simulink model "P702_NI_SoftECU"  (R2019a)
settings: Solver=ode1  StartTime=0.0  StopTime=Inf  FixedStep=0.001  RelTol=1e-3  EnableMultiTasking=on
PreLoadFcn:
  | run '.\VeriStand_BlockSet\NIVeriStandAddPaths.m'
undefined symbols (not defined in the file or in its folder): magnitude
libraries: simulink x83, simulink_extras x1
(part 65 of 76)

== system P702_NI_SoftECU/Output/Subsystem1/CAN_Signal/ECM_DIESEL PCM PCM_HEV/EngBrakeData_0x165 ==
  in_port : Inport
  AccEngStat_D_Actl : Terminator
  AccStopMde_D_Rq : Terminator
  BPedDrvAppl_D_QF : Terminator
  BpedDrvAppl_D_Actl : Terminator
  CcMde_D_Actl : Terminator
  CcOvrrdActv_B_Actl : Terminator
  CcStat_D_Actl : Terminator
  CmbbDeny_B_ActlPrpl : Terminator
  CmbbEngTqMn_B_Actl : Terminator
  EngAout_N_MnAllw : Terminator
  PrplTqMnSat_B_Actl : Terminator
  Veh_V_DsplyCcSet : Terminator
  bus_selector : BusSelector  OutputSignals=CmbbEngTqMn_B_Actl,CcOvrrdActv_B_Actl,BpedDrvAppl_D_Actl,CmbbDeny_B_ActlPrpl,AccEngStat_D_Actl,BPedDrvAppl_D_QF,CcMde_D_Actl,CcStat_D_Actl,Veh_V_DsplyCcSet,AccStopMde_D_Rq,PrplTqMnSat_B_Actl,EngAout_N_MnAllw
  wires:
  in_port/1 -> bus_selector/1  "Subsystem1"
  bus_selector/1 -> CmbbEngTqMn_B_Actl/1  "<CmbbEngTqMn_B_Actl>"
  bus_selector/2 -> CcOvrrdActv_B_Actl/1  "<CcOvrrdActv_B_Actl>"
  bus_selector/3 -> BpedDrvAppl_D_Actl/1  "<BpedDrvAppl_D_Actl>"
  bus_selector/4 -> CmbbDeny_B_ActlPrpl/1  "<CmbbDeny_B_ActlPrpl>"
  bus_selector/5 -> AccEngStat_D_Actl/1  "<AccEngStat_D_Actl>"
  bus_selector/6 -> BPedDrvAppl_D_QF/1  "<BPedDrvAppl_D_QF>"
  bus_selector/7 -> CcMde_D_Actl/1  "<CcMde_D_Actl>"
  bus_selector/8 -> CcStat_D_Actl/1  "<CcStat_D_Actl>"
  bus_selector/9 -> Veh_V_DsplyCcSet/1  "<Veh_V_DsplyCcSet>"
  bus_selector/10 -> AccStopMde_D_Rq/1  "<AccStopMde_D_Rq>"
  bus_selector/11 -> PrplTqMnSat_B_Actl/1  "<PrplTqMnSat_B_Actl>"
  bus_selector/12 -> EngAout_N_MnAllw/1  "<EngAout_N_MnAllw>"

== system P702_NI_SoftECU/Output/Subsystem1/CAN_Signal/ECM_DIESEL PCM PCM_HEV/EngVehicleSpThrottle2_0x202 ==
  in_port : Inport
  GearRvrse_D_Actl : Terminator
  StrtrMtrCtlMsgTxt_D2_Rq : Terminator
  StrtrMtrCtlMsgTxt_D_Rq : Terminator
  StrtrMtrDlyStrt_B_Stat : Terminator
  VehVActlEng_D_Qf : Terminator
  VehVActlEng_No_Cnt : Terminator
  VehVActlEng_No_Cs : Terminator
  VehVTrlrAid_B_Avail : Terminator
  Veh_V_ActlEng : Terminator
  Veh_V_RqCcSet : Terminator
  bus_selector : BusSelector  OutputSignals=StrtrMtrCtlMsgTxt_D_Rq,GearRvrse_D_Actl,StrtrMtrCtlMsgTxt_D2_Rq,VehVActlEng_No_Cs,VehVTrlrAid_B_Avail,VehVActlEng_No_Cnt,StrtrMtrDlyStrt_B_Stat,VehVActlEng_D_Qf,Veh_V_RqCcSet,Veh_V_ActlEng
  wires:
  in_port/1 -> bus_selector/1  "Subsystem1"
  bus_selector/1 -> StrtrMtrCtlMsgTxt_D_Rq/1  "<StrtrMtrCtlMsgTxt_D_Rq>"
  bus_selector/2 -> GearRvrse_D_Actl/1  "<GearRvrse_D_Actl>"
  bus_selector/3 -> StrtrMtrCtlMsgTxt_D2_Rq/1  "<StrtrMtrCtlMsgTxt_D2_Rq>"
  bus_selector/4 -> VehVActlEng_No_Cs/1  "<VehVActlEng_No_Cs>"
  bus_selector/5 -> VehVTrlrAid_B_Avail/1  "<VehVTrlrAid_B_Avail>"
  bus_selector/6 -> VehVActlEng_No_Cnt/1  "<VehVActlEng_No_Cnt>"
  bus_selector/7 -> StrtrMtrDlyStrt_B_Stat/1  "<StrtrMtrDlyStrt_B_Stat>"
  bus_selector/8 -> VehVActlEng_D_Qf/1  "<VehVActlEng_D_Qf>"
  bus_selector/9 -> Veh_V_RqCcSet/1  "<Veh_V_RqCcSet>"
  bus_selector/10 -> Veh_V_ActlEng/1  "<Veh_V_ActlEng>"

== system P702_NI_SoftECU/Output/Subsystem1/CAN_Signal/ECM_DIESEL PCM PCM_HEV/EngVehicleSpThrottle_0x204 ==
  in_port : Inport
  ApedPosPcActl_D_Qf : Terminator
  ApedPosPcActl_No_Cnt : Terminator
  ApedPosPcActl_No_Cs : Terminator
  ApedPos_PcRate_ActlArb : Terminator
  ApedPos_Pc_ActlArb : Terminator
  EngAout3_N_Actl : Terminator
  EngAoutNActl_D_QF : Terminator
  EngAout_N_Actl : Terminator
  bus_selector : BusSelector  OutputSignals=ApedPosPcActl_D_Qf,ApedPosPcActl_No_Cnt,ApedPos_Pc_ActlArb,ApedPos_PcRate_ActlArb,EngAoutNActl_D_QF,EngAout_N_Actl,ApedPosPcActl_No_Cs,EngAout3_N_Actl
  wires:
  in_port/1 -> bus_selector/1  "Subsystem1"
  bus_selector/1 -> ApedPosPcActl_D_Qf/1  "<ApedPosPcActl_D_Qf>"
  bus_selector/2 -> ApedPosPcActl_No_Cnt/1  "<ApedPosPcActl_No_Cnt>"
  bus_selector/3 -> ApedPos_Pc_ActlArb/1  "<ApedPos_Pc_ActlArb>"
  bus_selector/4 -> ApedPos_PcRate_ActlArb/1  "<ApedPos_PcRate_ActlArb>"
  bus_selector/5 -> EngAoutNActl_D_QF/1  "<EngAoutNActl_D_QF>"
  bus_selector/6 -> EngAout_N_Actl/1  "<EngAout_N_Actl>"
  bus_selector/7 -> ApedPosPcActl_No_Cs/1  "<ApedPosPcActl_No_Cs>"
  bus_selector/8 -> EngAout3_N_Actl/1  "<EngAout3_N_Actl>"

== system P702_NI_SoftECU/Output/Subsystem1/CAN_Signal/ECM_DIESEL PCM PCM_HEV/EngineClimateData_0x178 ==
  in_port : Inport
  AirAmbTe_D_Qf : Terminator
  AirAmb_P_Actl : Terminator
  AirAmb_Te_Actl : Terminator
  AirAmb_Te_ActlFilt : Terminator
  AslChime_B_Rq : Terminator
  AslIconDsply_D_Rq : Terminator
  DynoMde_B_Cmd : Terminator
  EcssLamp_D_RqDsply : Terminator
  EngAout_Aa_Actl : Terminator
  GasPrtc_D_RqDsply : Terminator
  HvacHtrCore2_Te_Actl : Terminator
  bus_selector : BusSelector  OutputSignals=DynoMde_B_Cmd,AslIconDsply_D_Rq,HvacHtrCore2_Te_Actl,GasPrtc_D_RqDsply,EcssLamp_D_RqDsply,EngAout_Aa_Actl,AslChime_B_Rq,AirAmbTe_D_Qf,AirAmb_Te_Actl,AirAmb_P_Actl,AirAmb_Te_ActlFilt
  wires:
  in_port/1 -> bus_selector/1  "Subsystem1"
  bus_selector/1 -> DynoMde_B_Cmd/1  "<DynoMde_B_Cmd>"
  bus_selector/2 -> AslIconDsply_D_Rq/1  "<AslIconDsply_D_Rq>"
  bus_selector/3 -> HvacHtrCore2_Te_Actl/1  "<HvacHtrCore2_Te_Actl>"
  bus_selector/4 -> GasPrtc_D_RqDsply/1  "<GasPrtc_D_RqDsply>"
  bus_selector/5 -> EcssLamp_D_RqDsply/1  "<EcssLamp_D_RqDsply>"
  bus_selector/6 -> EngAout_Aa_Actl/1  "<EngAout_Aa_Actl>"
  bus_selector/7 -> AslChime_B_Rq/1  "<AslChime_B_Rq>"
  bus_selector/8 -> AirAmbTe_D_Qf/1  "<AirAmbTe_D_Qf>"
  bus_selector/9 -> AirAmb_Te_Actl/1  "<AirAmb_Te_Actl>"
  bus_selector/10 -> AirAmb_P_Actl/1  "<AirAmb_P_Actl>"
  bus_selector/11 -> AirAmb_Te_ActlFilt/1  "<AirAmb_Te_ActlFilt>"

== system P702_NI_SoftECU/Output/Subsystem1/CAN_Signal/ECM_DIESEL PCM PCM_HEV/EngineData_6_0x156 ==
  in_port : Inport
  EngClntTe_D_Qf : Terminator
  EngClnt_Te_Actl : Terminator
  EngGoutLss_Tq_Est : Terminator
  EngOil_Te_Actl : Terminator
  EngOvrhtMitgActv_D_Ind : Terminator
  bus_selector : BusSelector  OutputSignals=EngClnt_Te_Actl,EngOil_Te_Actl,EngGoutLss_Tq_Est,EngOvrhtMitgActv_D_Ind,EngClntTe_D_Qf
  wires:
  in_port/1 -> bus_selector/1  "Subsystem1"
  bus_selector/1 -> EngClnt_Te_Actl/1  "<EngClnt_Te_Actl>"
  bus_selector/2 -> EngOil_Te_Actl/1  "<EngOil_Te_Actl>"
  bus_selector/3 -> EngGoutLss_Tq_Est/1  "<EngGoutLss_Tq_Est>"
  bus_selector/4 -> EngOvrhtMitgActv_D_Ind/1  "<EngOvrhtMitgActv_D_Ind>"
  bus_selector/5 -> EngClntTe_D_Qf/1  "<EngClntTe_D_Qf>"

== system P702_NI_SoftECU/Output/Subsystem1/CAN_Signal/ECM_DIESEL PCM PCM_HEV/EngineData_7_0x179 ==
  in_port : Inport
  AirCondClutch_B_Stats : Terminator
  AirCondRec_B_Rq : Terminator
  EngOilLife_Pc_Actl : Terminator
  EngSrvcRqd_B_Rq : Terminator
  FuelFillInlet_B_Dsply : Terminator
  FuelFilterLamp_B_Dsply : Terminator
  FuelFlw_Vl_Dsply : Terminator
  HvacAirFullOut_B_Rq : Terminator
  OdoCount : Terminator
  TrnKickDown_B_RqDrv : Terminator
  TrnManShifGear_D_IndDrv : Terminator
  TrnManShif_D_IndDrv : Terminator
  bus_selector : BusSelector  OutputSignals=TrnManShif_D_IndDrv,HvacAirFullOut_B_Rq,TrnKickDown_B_RqDrv,EngSrvcRqd_B_Rq,EngOilLife_Pc_Actl,FuelFillInlet_B_Dsply,OdoCount,AirCondRec_B_Rq,TrnManShifGear_D_IndDrv,AirCondClutch_B_Stats,FuelFilterLamp_B_Dsply,FuelFlw_Vl_Dsply
  wires:
  in_port/1 -> bus_selector/1  "Subsystem1"
  bus_selector/1 -> TrnManShif_D_IndDrv/1  "<TrnManShif_D_IndDrv>"
  bus_selector/2 -> HvacAirFullOut_B_Rq/1  "<HvacAirFullOut_B_Rq>"
  bus_selector/3 -> TrnKickDown_B_RqDrv/1  "<TrnKickDown_B_RqDrv>"
  bus_selector/4 -> EngSrvcRqd_B_Rq/1  "<EngSrvcRqd_B_Rq>"
  bus_selector/5 -> EngOilLife_Pc_Actl/1  "<EngOilLife_Pc_Actl>"
  bus_selector/6 -> FuelFillInlet_B_Dsply/1  "<FuelFillInlet_B_Dsply>"
  bus_selector/7 -> OdoCount/1  "<OdoCount>"
  bus_selector/8 -> AirCondRec_B_Rq/1  "<AirCondRec_B_Rq>"
  bus_selector/9 -> TrnManShifGear_D_IndDrv/1  "<TrnManShifGear_D_IndDrv>"
  bus_selector/10 -> AirCondClutch_B_Stats/1  "<AirCondClutch_B_Stats>"
  bus_selector/11 -> FuelFilterLamp_B_Dsply/1  "<FuelFilterLamp_B_Dsply>"
  bus_selector/12 -> FuelFlw_Vl_Dsply/1  "<FuelFlw_Vl_Dsply>"

== system P702_NI_SoftECU/Output/Subsystem1/CAN_Signal/ECM_DIESEL PCM PCM_HEV/Engine_Clutch_Data_0x42F ==
  in_port : Inport
  CluPdlPosPcMeas_D_Qf : Terminator
  CluPdlPos_Pc_Meas : Terminator
  CluPdl_PcRate_Actl : Terminator
  EngAoutIdl_N_Ntrl : Terminator
  EngAout_N_Dsply : Terminator
  bus_selector : BusSelector  OutputSignals=CluPdl_PcRate_Actl,CluPdlPosPcMeas_D_Qf,CluPdlPos_Pc_Meas,EngAoutIdl_N_Ntrl,EngAout_N_Dsply
  wires:
  in_port/1 -> bus_selector/1  "Subsystem1"
  bus_selector/1 -> CluPdl_PcRate_Actl/1  "<CluPdl_PcRate_Actl>"
  bus_selector/2 -> CluPdlPosPcMeas_D_Qf/1  "<CluPdlPosPcMeas_D_Qf>"
  bus_selector/3 -> CluPdlPos_Pc_Meas/1  "<CluPdlPos_Pc_Meas>"
  bus_selector/4 -> EngAoutIdl_N_Ntrl/1  "<EngAoutIdl_N_Ntrl>"
  bus_selector/5 -> EngAout_N_Dsply/1  "<EngAout_N_Dsply>"

== system P702_NI_SoftECU/Output/Subsystem1/CAN_Signal/ECM_DIESEL PCM PCM_HEV/Gear_Shift_by_Wire_3 ==
  in_port : Inport
  GearSelLck_D_Rq : Terminator
  PrkBrkActv_D_RqTrnGear : Terminator
  TrnCmdCnt_B_Actl : Terminator
  TrnCmdState_B_Actl : Terminator
  TrnDtpCmd_D_Actl : Terminator
  TrnGearCmd_No_Cnt : Terminator
  TrnGearCmd_No_Cs : Terminator
  TrnGearCmd_Pc_ActlPt : Terminator
  TrnGearMsgTxt_D_Rq : Terminator
  TrnGearNtmAllow_B_Stat : Terminator
  TrnGear_D_RqPt : Terminator
  TrnLvrV_D_Rq : Terminator
  TrnNtrlTowCmd_D_Actl : Terminator
  TrnSbwSysHlth_D_Actl : Terminator
  TrnValidGear_D_Cnfm : Terminator
  bus_selector : BusSelector  OutputSignals=GearSelLck_D_Rq,PrkBrkActv_D_RqTrnGear,TrnCmdCnt_B_Actl,TrnCmdState_B_Actl,TrnDtpCmd_D_Actl,TrnGearCmd_No_Cnt,TrnGearCmd_No_Cs,TrnGearCmd_Pc_ActlPt,TrnGearMsgTxt_D_Rq,TrnGearNtmAllow_B_Stat,TrnGear_D_RqPt,TrnLvrV_D_Rq,TrnNtrlTowCmd_D_Actl,TrnSbwSysHlth_D_Actl,TrnValidGear_D_Cnfm
  wires:
  in_port/1 -> bus_selector/1  "Subsystem1"
  bus_selector/1 -> GearSelLck_D_Rq/1  "<GearSelLck_D_Rq>"
  bus_selector/2 -> PrkBrkActv_D_RqTrnGear/1  "<PrkBrkActv_D_RqTrnGear>"
  bus_selector/3 -> TrnCmdCnt_B_Actl/1  "<TrnCmdCnt_B_Actl>"
  bus_selector/4 -> TrnCmdState_B_Actl/1  "<TrnCmdState_B_Actl>"
  bus_selector/5 -> TrnDtpCmd_D_Actl/1  "<TrnDtpCmd_D_Actl>"
  bus_selector/6 -> TrnGearCmd_No_Cnt/1  "<TrnGearCmd_No_Cnt>"
  bus_selector/7 -> TrnGearCmd_No_Cs/1  "<TrnGearCmd_No_Cs>"
  bus_selector/8 -> TrnGearCmd_Pc_ActlPt/1  "<TrnGearCmd_Pc_ActlPt>"
  bus_selector/9 -> TrnGearMsgTxt_D_Rq/1  "<TrnGearMsgTxt_D_Rq>"
  bus_selector/10 -> TrnGearNtmAllow_B_Stat/1  "<TrnGearNtmAllow_B_Stat>"
  bus_selector/11 -> TrnGear_D_RqPt/1  "<TrnGear_D_RqPt>"
  bus_selector/12 -> TrnLvrV_D_Rq/1  "<TrnLvrV_D_Rq>"
  bus_selector/13 -> TrnNtrlTowCmd_D_Actl/1  "<TrnNtrlTowCmd_D_Actl>"
  bus_selector/14 -> TrnSbwSysHlth_D_Actl/1  "<TrnSbwSysHlth_D_Actl>"
  bus_selector/15 -> TrnValidGear_D_Cnfm/1  "<TrnValidGear_D_Cnfm>"

== system P702_NI_SoftECU/Output/Subsystem1/CAN_Signal/ECM_DIESEL PCM PCM_HEV/Global_PATS_TargetInfo_0x47 ==
  in_port : Inport
  bus_selector : BusSelector  OutputSignals=immoTarget1Status,immoTarget1Cmd,immoTarget1Data
  immoTarget1Cmd : Terminator
  immoTarget1Data : Terminator
  immoTarget1Status : Terminator
  wires:
  in_port/1 -> bus_selector/1  "Subsystem1"
  bus_selector/1 -> immoTarget1Status/1  "<immoTarget1Status>"
  bus_selector/2 -> immoTarget1Cmd/1  "<immoTarget1Cmd>"
  bus_selector/3 -> immoTarget1Data/1  "<immoTarget1Data>"

== system P702_NI_SoftECU/Output/Subsystem1/CAN_Signal/ECM_DIESEL PCM PCM_HEV/HEV_Powertrain_Data2 ==
  in_port : Inport
  BattTracCnnct_D_Rq : Terminator
  PrplTqMnRgen_B_Actl : Terminator
  WhlDirAvgDrv_D_Actl : Terminator
  bus_selector : BusSelector  OutputSignals=BattTracCnnct_D_Rq,PrplTqMnRgen_B_Actl,WhlDirAvgDrv_D_Actl
  wires:
  in_port/1 -> bus_selector/1  "Subsystem1"
  bus_selector/1 -> BattTracCnnct_D_Rq/1  "<BattTracCnnct_D_Rq>"
  bus_selector/2 -> PrplTqMnRgen_B_Actl/1  "<PrplTqMnRgen_B_Actl>"
  bus_selector/3 -> WhlDirAvgDrv_D_Actl/1  "<WhlDirAvgDrv_D_Actl>"

== system P702_NI_SoftECU/Output/Subsystem1/CAN_Signal/ECM_DIESEL PCM PCM_HEV/PCM_AutoSar_NetworkMgmt_0x595 ==
  in_port : Inport
  PCM_AutoSarNMControl : Terminator
  PCM_AutoSarNMNodeId : Terminator
  PCM_AutoSarNMReserved{1..4} (4 alike) : Terminator
  PCM_GWNMProxy : Terminator
  PCM_GWOnBoardTester : Terminator
  bus_selector : BusSelector  OutputSignals=PCM_AutoSarNMNodeId,PCM_AutoSarNMControl,PCM_AutoSarNMReserved1,PCM_AutoSarNMReserved2,PCM_GWOnBoardTester,PCM_GWNMProxy,PCM_AutoSarNMReserved3,PCM_AutoSarNMReserved4
  wires:
  in_port/1 -> bus_selector/1  "Subsystem1"
  bus_selector/1 -> PCM_AutoSarNMNodeId/1  "<PCM_AutoSarNMNodeId>"
  bus_selector/2 -> PCM_AutoSarNMControl/1  "<PCM_AutoSarNMControl>"
  bus_selector/3 -> PCM_AutoSarNMReserved1/1  "<PCM_AutoSarNMReserved1>"
  bus_selector/4 -> PCM_AutoSarNMReserved2/1  "<PCM_AutoSarNMReserved2>"
  bus_selector/5 -> PCM_GWOnBoardTester/1  "<PCM_GWOnBoardTester>"
  bus_selector/6 -> PCM_GWNMProxy/1  "<PCM_GWNMProxy>"
  bus_selector/7 -> PCM_AutoSarNMReserved3/1  "<PCM_AutoSarNMReserved3>"
  bus_selector/8 -> PCM_AutoSarNMReserved4/1  "<PCM_AutoSarNMReserved4>"

== system P702_NI_SoftECU/Output/Subsystem1/CAN_Signal/ECM_DIESEL PCM PCM_HEV/PCM_Rapid_Data_Response_1_0x6A0 ==
  in_port : Inport
  UUDTPCMResponse1 : Terminator
  bus_selector : BusSelector  OutputSignals=UUDTPCMResponse1
  wires:
  in_port/1 -> bus_selector/1  "Subsystem1"
  bus_selector/1 -> UUDTPCMResponse1/1  "<UUDTPCMResponse1>"

== system P702_NI_SoftECU/Output/Subsystem1/CAN_Signal/ECM_DIESEL PCM PCM_HEV/PowertrainData_10 ==
  in_port : Inport
  GearEngag_D_Actl : Terminator
  GearLvr_D_ActlDrv : Terminator
  GearPos_D_Actl : Terminator
  GearPos_D_Trg : Terminator
  GearPos_No_Cnt : Terminator
  GearPos_No_Cs : Terminator
  TrnIgnOffDly_T_Rq : Terminator
  TrnPrkSys_D_Actl : Terminator
  TrnRng_D_Rq : Terminator
  bus_selector : BusSelector  OutputSignals=GearEngag_D_Actl,GearLvr_D_ActlDrv,GearPos_D_Actl,GearPos_D_Trg,GearPos_No_Cnt,GearPos_No_Cs,TrnIgnOffDly_T_Rq,TrnPrkSys_D_Actl,TrnRng_D_Rq
  wires:
  in_port/1 -> bus_selector/1  "Subsystem1"
  bus_selector/1 -> GearEngag_D_Actl/1  "<GearEngag_D_Actl>"
  bus_selector/2 -> GearLvr_D_ActlDrv/1  "<GearLvr_D_ActlDrv>"
  bus_selector/3 -> GearPos_D_Actl/1  "<GearPos_D_Actl>"
  bus_selector/4 -> GearPos_D_Trg/1  "<GearPos_D_Trg>"
  bus_selector/5 -> GearPos_No_Cnt/1  "<GearPos_No_Cnt>"
  bus_selector/6 -> GearPos_No_Cs/1  "<GearPos_No_Cs>"
  bus_selector/7 -> TrnIgnOffDly_T_Rq/1  "<TrnIgnOffDly_T_Rq>"
  bus_selector/8 -> TrnPrkSys_D_Actl/1  "<TrnPrkSys_D_Actl>"
  bus_selector/9 -> TrnRng_D_Rq/1  "<TrnRng_D_Rq>"

== system P702_NI_SoftECU/Output/Subsystem1/CAN_Signal/ECM_DIESEL PCM PCM_HEV/PowertrainData_1_0x421 ==
  in_port : Inport
  AirCondFluidHi_P_Actl : Terminator
  CoolantFanStepAct : Terminator
  ECMMILRequest : Terminator
  EngIdlShutDown_D_Stat : Terminator
  EngIdlShutDwnTxt_D_Rq : Terminator
  FUEL_ALCOHOL_PERCNT : Terminator
  FohEng_D_Rq : Terminator
  OilPressureWarning : Terminator
  TrnTotLss_Tq_Est : Terminator
  TrnTotTq_Rt_Est : Terminator
  VehVLimActv_B_Actl : Terminator
  VehVLimStat_D_Actl : Terminator
  bus_selector : BusSelector  OutputSignals=VehVLimActv_B_Actl,VehVLimStat_D_Actl,ECMMILRequest,FohEng_D_Rq,EngIdlShutDown_D_Stat,CoolantFanStepAct,OilPressureWarning,EngIdlShutDwnTxt_D_Rq,TrnTotLss_Tq_Est,TrnTotTq_Rt_Est,AirCondFluidHi_P_Actl,FUEL_ALCOHOL_PERCNT
  wires:
  in_port/1 -> bus_selector/1  "Subsystem1"
  bus_selector/1 -> VehVLimActv_B_Actl/1  "<VehVLimActv_B_Actl>"
  bus_selector/2 -> VehVLimStat_D_Actl/1  "<VehVLimStat_D_Actl>"
  bus_selector/3 -> ECMMILRequest/1  "<ECMMILRequest>"
  bus_selector/4 -> FohEng_D_Rq/1  "<FohEng_D_Rq>"
  bus_selector/5 -> EngIdlShutDown_D_Stat/1  "<EngIdlShutDown_D_Stat>"
  bus_selector/6 -> CoolantFanStepAct/1  "<CoolantFanStepAct>"
  bus_selector/7 -> OilPressureWarning/1  "<OilPressureWarning>"
  bus_selector/8 -> EngIdlShutDwnTxt_D_Rq/1  "<EngIdlShutDwnTxt_D_Rq>"
  bus_selector/9 -> TrnTotLss_Tq_Est/1  "<TrnTotLss_Tq_Est>"
  bus_selector/10 -> TrnTotTq_Rt_Est/1  "<TrnTotTq_Rt_Est>"
  bus_selector/11 -> AirCondFluidHi_P_Actl/1  "<AirCondFluidHi_P_Actl>"
  bus_selector/12 -> FUEL_ALCOHOL_PERCNT/1  "<FUEL_ALCOHOL_PERCNT>"

== system P702_NI_SoftECU/Output/Subsystem1/CAN_Signal/ECM_DIESEL PCM PCM_HEV/PowertrainData_2_0x42D ==
  in_port : Inport
  ApedPos_Pc_ActlDiag : Terminator
  EngAirIn_Te_Actl : Terminator
  EngClnt_Te_ActlDiag : Terminator
  EngLoad_Pc_CalcDiag : Terminator
  EngMsgTxt_D_Rq : Terminator
  GrllShtrPos_B_Falt : Terminator
  GrllShtrPos_D_Cmd : Terminator
  IsaOffst_D_Stat : Terminator
  ObdWarmUp_B_Complt : Terminator
  SlMde_D_RqDsply : Terminator
  SlMde_D_Stat : Terminator
  bus_selector : BusSelector  OutputSignals=ObdWarmUp_B_Complt,EngMsgTxt_D_Rq,EngAirIn_Te_Actl,ApedPos_Pc_ActlDiag,EngClnt_Te_ActlDiag,EngLoad_Pc_CalcDiag,GrllShtrPos_D_Cmd,GrllShtrPos_B_Falt,IsaOffst_D_Stat,SlMde_D_RqDsply,SlMde_D_Stat
  wires:
  in_port/1 -> bus_selector/1  "Subsystem1"
  bus_selector/1 -> ObdWarmUp_B_Complt/1  "<ObdWarmUp_B_Complt>"
  bus_selector/2 -> EngMsgTxt_D_Rq/1  "<EngMsgTxt_D_Rq>"
  bus_selector/3 -> EngAirIn_Te_Actl/1  "<EngAirIn_Te_Actl>"
  bus_selector/4 -> ApedPos_Pc_ActlDiag/1  "<ApedPos_Pc_ActlDiag>"
  bus_selector/5 -> EngClnt_Te_ActlDiag/1  "<EngClnt_Te_ActlDiag>"
  bus_selector/6 -> EngLoad_Pc_CalcDiag/1  "<EngLoad_Pc_CalcDiag>"
  bus_selector/7 -> GrllShtrPos_D_Cmd/1  "<GrllShtrPos_D_Cmd>"
  bus_selector/8 -> GrllShtrPos_B_Falt/1  "<GrllShtrPos_B_Falt>"
  bus_selector/9 -> IsaOffst_D_Stat/1  "<IsaOffst_D_Stat>"
  bus_selector/10 -> SlMde_D_RqDsply/1  "<SlMde_D_RqDsply>"
  bus_selector/11 -> SlMde_D_Stat/1  "<SlMde_D_Stat>"

== system P702_NI_SoftECU/Output/Subsystem1/CAN_Signal/ECM_DIESEL PCM PCM_HEV/PowertrainData_3_0x43E ==
  in_port : Inport
  BattULoChrg_U_Cmd : Terminator
  ElLoadCtl_D_Rq : Terminator
  EngMnfld_P_Actl : Terminator
  FuelPumpPwr_B_Rq : Terminator
  bus_selector : BusSelector  OutputSignals=BattULoChrg_U_Cmd,ElLoadCtl_D_Rq,FuelPumpPwr_B_Rq,EngMnfld_P_Actl
  wires:
  in_port/1 -> bus_selector/1  "Subsystem1"
  bus_selector/1 -> BattULoChrg_U_Cmd/1  "<BattULoChrg_U_Cmd>"
  bus_selector/2 -> ElLoadCtl_D_Rq/1  "<ElLoadCtl_D_Rq>"
  bus_selector/3 -> FuelPumpPwr_B_Rq/1  "<FuelPumpPwr_B_Rq>"
  bus_selector/4 -> EngMnfld_P_Actl/1  "<EngMnfld_P_Actl>"

== system P702_NI_SoftECU/Output/Subsystem1/CAN_Signal/ECM_DIESEL PCM PCM_HEV/PowertrainData_6_0x205 ==
  in_port : Inport
  BrkTot_Tq_RqFapLc : Terminator
  FapLc_B_Err : Terminator
  TrnAin_Pc_RqDrv : Terminator
  bus_selector : BusSelector  OutputSignals=BrkTot_Tq_RqFapLc,FapLc_B_Err,TrnAin_Pc_RqDrv
  wires:
  in_port/1 -> bus_selector/1  "Subsystem1"
  bus_selector/1 -> BrkTot_Tq_RqFapLc/1  "<BrkTot_Tq_RqFapLc>"
  bus_selector/2 -> FapLc_B_Err/1  "<FapLc_B_Err>"
  bus_selector/3 -> TrnAin_Pc_RqDrv/1  "<TrnAin_Pc_RqDrv>"

== system P702_NI_SoftECU/Output/Subsystem1/CAN_Signal/ECM_DIESEL PCM PCM_HEV/PowertrainData_7_0x41F ==
  in_port : Inport
  EcoCochA_Pc_Dsply : Terminator
  EcoCochCrus_Pc_Dsply : Terminator
  EcoCochDecel_Pc_Dsply : Terminator
  EcoCochIdlFuel_Pc_Dsply : Terminator
  EcoCochInstNeg_B_Dsply : Terminator
  EcoCochInst_Pc_Dsply : Terminator
  EcoCochShif_Pc_Dsply : Terminator
  bus_selector : BusSelector  OutputSignals=EcoCochA_Pc_Dsply,EcoCochCrus_Pc_Dsply,EcoCochDecel_Pc_Dsply,EcoCochIdlFuel_Pc_Dsply,EcoCochShif_Pc_Dsply,EcoCochInst_Pc_Dsply,EcoCochInstNeg_B_Dsply
  wires:
  in_port/1 -> bus_selector/1  "Subsystem1"
  bus_selector/1 -> EcoCochA_Pc_Dsply/1  "<EcoCochA_Pc_Dsply>"
  bus_selector/2 -> EcoCochCrus_Pc_Dsply/1  "<EcoCochCrus_Pc_Dsply>"
  bus_selector/3 -> EcoCochDecel_Pc_Dsply/1  "<EcoCochDecel_Pc_Dsply>"
  bus_selector/4 -> EcoCochIdlFuel_Pc_Dsply/1  "<EcoCochIdlFuel_Pc_Dsply>"
  bus_selector/5 -> EcoCochShif_Pc_Dsply/1  "<EcoCochShif_Pc_Dsply>"
  bus_selector/6 -> EcoCochInst_Pc_Dsply/1  "<EcoCochInst_Pc_Dsply>"
  bus_selector/7 -> EcoCochInstNeg_B_Dsply/1  "<EcoCochInstNeg_B_Dsply>"

== system P702_NI_SoftECU/Output/Subsystem1/CAN_Signal/ECM_DIESEL PCM PCM_HEV/PowertrainData_9_0x44C ==
  in_port : Inport
  AutoTowActv_B_Stat : Terminator
  AutoTowAllw_D_StatMnu : Terminator
  GrossTrainWeight_M_Est : Terminator
  TrailCtlPt_B_Falt : Terminator
  Veh_V_DsplyTrailCtlSet : Terminator
  WakeAlarm1_B_Typ : Terminator
  WakeAlarm1_T_Rq : Terminator
  bus_selector : BusSelector  OutputSignals=GrossTrainWeight_M_Est,AutoTowAllw_D_StatMnu,AutoTowActv_B_Stat,TrailCtlPt_B_Falt,Veh_V_DsplyTrailCtlSet,WakeAlarm1_T_Rq,WakeAlarm1_B_Typ
  wires:
  in_port/1 -> bus_selector/1  "Subsystem1"
  bus_selector/1 -> GrossTrainWeight_M_Est/1  "<GrossTrainWeight_M_Est>"
  bus_selector/2 -> AutoTowAllw_D_StatMnu/1  "<AutoTowAllw_D_StatMnu>"
  bus_selector/3 -> AutoTowActv_B_Stat/1  "<AutoTowActv_B_Stat>"
  bus_selector/4 -> TrailCtlPt_B_Falt/1  "<TrailCtlPt_B_Falt>"
  bus_selector/5 -> Veh_V_DsplyTrailCtlSet/1  "<Veh_V_DsplyTrailCtlSet>"
  bus_selector/6 -> WakeAlarm1_T_Rq/1  "<WakeAlarm1_T_Rq>"
  bus_selector/7 -> WakeAlarm1_B_Typ/1  "<WakeAlarm1_B_Typ>"

== system P702_NI_SoftECU/Output/Subsystem1/CAN_Signal/ECM_DIESEL PCM PCM_HEV/Powertrain_Data_4_0x424 ==
  in_port : Inport
  BpedDrvMsgTxt_B_Dsply : Terminator
  FuelLvlWarn_D_ActlEng : Terminator
  FuelLvl_Pc_DsplyEng : Terminator
  FuelRange_L_DsplyEng : Terminator
  RearDiffOilTeWarn_B_Rq : Terminator
  RearDiffOil_Te_Actl : Terminator
  SelDrvMdePt_D_Stat : Terminator
  bus_selector : BusSelector  OutputSignals=BpedDrvMsgTxt_B_Dsply,RearDiffOil_Te_Actl,RearDiffOilTeWarn_B_Rq,FuelLvlWarn_D_ActlEng,SelDrvMdePt_D_Stat,FuelRange_L_DsplyEng,FuelLvl_Pc_DsplyEng
  wires:
  in_port/1 -> bus_selector/1  "Subsystem1"
  bus_selector/1 -> BpedDrvMsgTxt_B_Dsply/1  "<BpedDrvMsgTxt_B_Dsply>"
  bus_selector/2 -> RearDiffOil_Te_Actl/1  "<RearDiffOil_Te_Actl>"
  bus_selector/3 -> RearDiffOilTeWarn_B_Rq/1  "<RearDiffOilTeWarn_B_Rq>"
  bus_selector/4 -> FuelLvlWarn_D_ActlEng/1  "<FuelLvlWarn_D_ActlEng>"
  bus_selector/5 -> SelDrvMdePt_D_Stat/1  "<SelDrvMdePt_D_Stat>"
  bus_selector/6 -> FuelRange_L_DsplyEng/1  "<FuelRange_L_DsplyEng>"
  bus_selector/7 -> FuelLvl_Pc_DsplyEng/1  "<FuelLvl_Pc_DsplyEng>"

== system P702_NI_SoftECU/Output/Subsystem1/CAN_Signal/ECM_DIESEL PCM PCM_HEV/Powertrain_Data_5_0x43F ==
  in_port : Inport
  FapLcActv_B_Stat : Terminator
  FapLcInhbt_B_Rq : Terminator
  FapLcMaxGrdAbrt_B_Stat : Terminator
  FapLcMaxGrdInhbt_B_Stat : Terminator
  FapLcObstcl_B_Stat : Terminator
  FapLcPrchgBrk_B_Rq : Terminator
  FapLcStopHold_B_Rq : Terminator
  bus_selector : BusSelector  OutputSignals=FapLcActv_B_Stat,FapLcMaxGrdAbrt_B_Stat,FapLcMaxGrdInhbt_B_Stat,FapLcObstcl_B_Stat,FapLcPrchgBrk_B_Rq,FapLcStopHold_B_Rq,FapLcInhbt_B_Rq
  wires:
  in_port/1 -> bus_selector/1  "Subsystem1"
  bus_selector/1 -> FapLcActv_B_Stat/1  "<FapLcActv_B_Stat>"
  bus_selector/2 -> FapLcMaxGrdAbrt_B_Stat/1  "<FapLcMaxGrdAbrt_B_Stat>"
  bus_selector/3 -> FapLcMaxGrdInhbt_B_Stat/1  "<FapLcMaxGrdInhbt_B_Stat>"
  bus_selector/4 -> FapLcObstcl_B_Stat/1  "<FapLcObstcl_B_Stat>"
  bus_selector/5 -> FapLcPrchgBrk_B_Rq/1  "<FapLcPrchgBrk_B_Rq>"
  bus_selector/6 -> FapLcStopHold_B_Rq/1  "<FapLcStopHold_B_Rq>"
  bus_selector/7 -> FapLcInhbt_B_Rq/1  "<FapLcInhbt_B_Rq>"

== system P702_NI_SoftECU/Output/Subsystem1/CAN_Signal/ECM_DIESEL PCM PCM_HEV/Stop_Start_0x166 ==
  in_port : Inport
  AutoStopPtDelta_I_Est : Terminator
  HiElPwInhbt_B_Stat : Terminator
  OdoTripVerify_L_Actl : Terminator
  StopStrtDrvMde_D_Indic : Terminator
  StopStrtIODTxt_D_Rq : Terminator
  StopStrtMsgTxt_D_Rq : Terminator
  StopStrtStdby_D_Indic : Terminator
  bus_selector : BusSelector  OutputSignals=AutoStopPtDelta_I_Est,HiElPwInhbt_B_Stat,StopStrtDrvMde_D_Indic,StopStrtMsgTxt_D_Rq,OdoTripVerify_L_Actl,StopStrtStdby_D_Indic,StopStrtIODTxt_D_Rq
  wires:
  in_port/1 -> bus_selector/1  "Subsystem1"
  bus_selector/1 -> AutoStopPtDelta_I_Est/1  "<AutoStopPtDelta_I_Est>"
  bus_selector/2 -> HiElPwInhbt_B_Stat/1  "<HiElPwInhbt_B_Stat>"
  bus_selector/3 -> StopStrtDrvMde_D_Indic/1  "<StopStrtDrvMde_D_Indic>"
  bus_selector/4 -> StopStrtMsgTxt_D_Rq/1  "<StopStrtMsgTxt_D_Rq>"
  bus_selector/5 -> OdoTripVerify_L_Actl/1  "<OdoTripVerify_L_Actl>"
  bus_selector/6 -> StopStrtStdby_D_Indic/1  "<StopStrtStdby_D_Indic>"
  bus_selector/7 -> StopStrtIODTxt_D_Rq/1  "<StopStrtIODTxt_D_Rq>"

== system P702_NI_SoftECU/Output/Subsystem1/CAN_Signal/ECM_DIESEL PCM PCM_HEV/TesterPhysicalResPCM_0x7E8 ==
  in_port : Inport
  TesterPhysicalResPCM : Terminator
  bus_selector : BusSelector  OutputSignals=TesterPhysicalResPCM
  wires:
  in_port/1 -> bus_selector/1  "Subsystem1"
  bus_selector/1 -> TesterPhysicalResPCM/1  "<TesterPhysicalResPCM>"

== system P702_NI_SoftECU/Output/Subsystem1/CAN_Signal/ECM_DIESEL PCM PCM_HEV/TorqueDataEngFlags_0x200 ==
  in_port : Inport
  PrplWhlTotTqRq_No_Cnt : Terminator
  PrplWhlTotTqRq_No_Cs : Terminator
  PrplWhlTot_Tq_LimMn : Terminator
  PrplWhlTot_Tq_Rq : Terminator
  PtDrvMde_D_Stat : Terminator
  bus_selector : BusSelector  OutputSignals=PrplWhlTot_Tq_LimMn,PrplWhlTot_Tq_Rq,PtDrvMde_D_Stat,PrplWhlTotTqRq_No_Cnt,PrplWhlTotTqRq_No_Cs
  wires:
  in_port/1 -> bus_selector/1  "Subsystem1"
  bus_selector/1 -> PrplWhlTot_Tq_LimMn/1  "<PrplWhlTot_Tq_LimMn>"
  bus_selector/2 -> PrplWhlTot_Tq_Rq/1  "<PrplWhlTot_Tq_Rq>"
  bus_selector/3 -> PtDrvMde_D_Stat/1  "<PtDrvMde_D_Stat>"
  bus_selector/4 -> PrplWhlTotTqRq_No_Cnt/1  "<PrplWhlTotTqRq_No_Cnt>"
  bus_selector/5 -> PrplWhlTotTqRq_No_Cs/1  "<PrplWhlTotTqRq_No_Cs>"

== system P702_NI_SoftECU/Output/Subsystem1/CAN_Signal/ECM_DIESEL PCM PCM_HEV/TransGearData ==
  in_port : Inport
  GboxOil_Te_Actl : Terminator
  GearLvrPos_D_Actl : Terminator
  SelDrvMdeSwtch_D_Stat3 : Terminator
  TrnShifActv_B_Actl : Terminator
  TrnSrvcRqd_B_Rq : Terminator
  bus_selector : BusSelector  OutputSignals=GboxOil_Te_Actl,GearLvrPos_D_Actl,SelDrvMdeSwtch_D_Stat3,TrnShifActv_B_Actl,TrnSrvcRqd_B_Rq
  wires:
  in_port/1 -> bus_selector/1  "Subsystem1"
  bus_selector/1 -> GboxOil_Te_Actl/1  "<GboxOil_Te_Actl>"
  bus_selector/2 -> GearLvrPos_D_Actl/1  "<GearLvrPos_D_Actl>"
  bus_selector/3 -> SelDrvMdeSwtch_D_Stat3/1  "<SelDrvMdeSwtch_D_Stat3>"
  bus_selector/4 -> TrnShifActv_B_Actl/1  "<TrnShifActv_B_Actl>"
  bus_selector/5 -> TrnSrvcRqd_B_Rq/1  "<TrnSrvcRqd_B_Rq>"

== system P702_NI_SoftECU/Output/Subsystem1/CAN_Signal/ECM_DIESEL PCM PCM_HEV/VehicleOperatingModes_0x167 ==
  in_port : Inport
  ElPw_D_Stat : Terminator
  ElPw_D_StatStrtStop : Terminator
  Eng_D_Stat : Terminator
  PlgActvArb_B_Actl : Terminator
  PrplWhlRgenMn_Tq_Actl : Terminator
  PrplWhlTot2_Tq_Actl : Terminator
  PwPckTq_D_Stat : Terminator
  TrnAinTq_D_Qf : Terminator
  TrnAin_Tq_Actl : Terminator
  bus_selector : BusSelector  OutputSignals=Eng_D_Stat,PwPckTq_D_Stat,ElPw_D_Stat,PlgActvArb_B_Actl,PrplWhlTot2_Tq_Actl,ElPw_D_StatStrtStop,PrplWhlRgenMn_Tq_Actl,TrnAinTq_D_Qf,TrnAin_Tq_Actl
  wires:
  in_port/1 -> bus_selector/1  "Subsystem1"
  bus_selector/1 -> Eng_D_Stat/1  "<Eng_D_Stat>"
  bus_selector/2 -> PwPckTq_D_Stat/1  "<PwPckTq_D_Stat>"
  bus_selector/3 -> ElPw_D_Stat/1  "<ElPw_D_Stat>"
  bus_selector/4 -> PlgActvArb_B_Actl/1  "<PlgActvArb_B_Actl>"
  bus_selector/5 -> PrplWhlTot2_Tq_Actl/1  "<PrplWhlTot2_Tq_Actl>"
  bus_selector/6 -> ElPw_D_StatStrtStop/1  "<ElPw_D_StatStrtStop>"
  bus_selector/7 -> PrplWhlRgenMn_Tq_Actl/1  "<PrplWhlRgenMn_Tq_Actl>"
  bus_selector/8 -> TrnAinTq_D_Qf/1  "<TrnAinTq_D_Qf>"
  bus_selector/9 -> TrnAin_Tq_Actl/1  "<TrnAin_Tq_Actl>"

== system P702_NI_SoftECU/Output/Subsystem1/CAN_Signal/GWM/GSM ==
  in_port : Inport
  Gear_Shift_by_Wire_2_FD1_168 : Subsystem
  Gear_Shift_by_Wire_FD1_5A : Subsystem
  bus_selector : BusSelector  OutputSignals=Gear_Shift_by_Wire_2_FD1_168,Gear_Shift_by_Wire_FD1_5A
  wires:
  in_port/1 -> bus_selector/1  "Subsystem1"
  bus_selector/1 -> Gear_Shift_by_Wire_2_FD1_168/1(in_port)  "<Gear_Shift_by_Wire_2_FD1_168>"
  bus_selector/2 -> Gear_Shift_by_Wire_FD1_5A/1(in_port)  "<Gear_Shift_by_Wire_FD1_5A>"

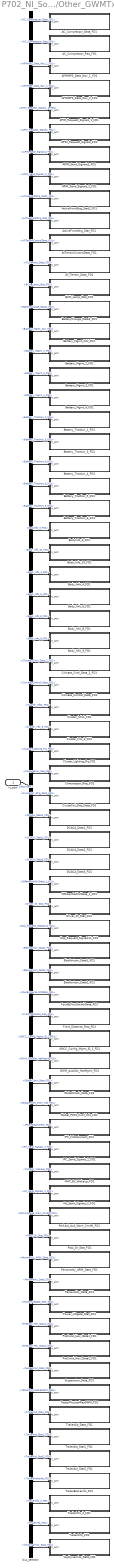
== system P702_NI_SoftECU/Output/Subsystem1/CAN_Signal/GWM/Other_GWMTx ==
  in_port : Inport
  AC_Compressor_Data_FD1 : Subsystem
  AC_Compressor_Req_FD1 : Subsystem
  APIMGPS_Data_Nav_1_FD1 : Subsystem
  APIMGPS_Data_Nav_2_FD1 : Subsystem
  APIM_Request_Signals_1_FD1 : Subsystem
  APIM_Request_Signals_FD1 : Subsystem
  APIM_Send_Signals1_FD1 : Subsystem
  APIM_Send_Signals_2_FD1 : Subsystem
  ActiveFrontStrg_Stat2_FD1 : Subsystem
  ActiveFrontStrg_Stat_FD1 : Subsystem
  AllTerrainControlData_FD1 : Subsystem
  All_Terrain_Data_FD1 : Subsystem
  BCM_Lamp_Stat_FD1 : Subsystem
  BatteryCharge_Data2_FD1 : Subsystem
  Battery_Mgmt_24V_FD1 : Subsystem
  Battery_Mgmt_2_FD1 : Subsystem
  Battery_Mgmt_3_FD1 : Subsystem
  Battery_Mgmt_4_FD1 : Subsystem
  Battery_Traction_1_FD1 : Subsystem
  Battery_Traction_3_FD1 : Subsystem
  Battery_Traction_4_FD1 : Subsystem
  Battery_Traction_5_FD1 : Subsystem
  Battery_Traction_6_FD1 : Subsystem
  BodyInfo_3_FD1 : Subsystem
  Body_Info_10_FD1 : Subsystem
  Body_Info_4_FD1 : Subsystem
  Body_Info_6_FD1 : Subsystem
  Body_Info_8_FD1 : Subsystem
  Body_Info_9_FD1 : Subsystem
  Climate_Cntrl_Data_2_FD1 : Subsystem
  Climate_Control_Data_FD1 : Subsystem
  Cluster_Info1_FD1 : Subsystem
  Cluster_Info_3_FD1 : Subsystem
  Cluster_Lighting_Rq_FD1 : Subsystem
  Compressor_Req_FD1 : Subsystem
  CruiseCtrl_Strg_Data_FD1 : Subsystem
  DCACA_Data1_FD1 : Subsystem
  DCACA_Data2_FD1 : Subsystem
  DCACA_Data3_FD1 : Subsystem
  DifferentialCtrlData_1_FD1 : Subsystem
  Driver_Dr_Stat_FD1 : Subsystem
  Dsp_Request_Signals11_FD1 : Subsystem
  ElecHorizon_Data1_FD1 : Subsystem
  ElecHorizon_Data2_FD1 : Subsystem
  FourByFourSwitchData_FD1 : Subsystem
  Front_Distance_Req_FD1 : Subsystem
  GGCC_Config_Mgmt_ID_1_FD1 : Subsystem
  GWM_AutoSar_NetMgmt_FD1 : Subsystem
  GlobalClock_Data_FD1 : Subsystem
  Global_PATS_Cntrl_Info_FD1 : Subsystem
  IPC_Infotainment_FD1 : Subsystem
  IPC_Send_Signals_2_FD1 : Subsystem
  MHT_EV_Wakeup_FD1 : Subsystem
  Mc_Send_Signals_2_FD1 : Subsystem
  ParkAid_Aud_Warn_CmdM_FD1 : Subsystem
  Pass_Dr_Stat_FD1 : Subsystem
  Personality_APIM_Data_FD1 : Subsystem
  Personality_Data_FD1 : Subsystem
  Power_Liftgate_Stat_FD1 : Subsystem
  PreCond_Hev_Data1_FD1 : Subsystem
  PreCond_Hev_Data2_FD1 : Subsystem
  Suspension_Data_FD1 : Subsystem
  TesterPhysicalResGWM_FD1 : Subsystem
  TrailerAid_Data_FD1 : Subsystem
  TrailerAid_Stat1_FD1 : Subsystem
  TrailerAid_Stat2_FD1 : Subsystem
  TrailerBrakeInfo_FD1 : Subsystem
  TrailerInfo_2_FD1 : Subsystem
  TrailerInfo_FD1 : Subsystem
  VeyDynamics_Data_FD1 : Subsystem
  bus_selector : BusSelector  OutputSignals=AC_Compressor_Data_FD1,AC_Compressor_Req_FD1,APIMGPS_Data_Nav_1_FD1,APIMGPS_Data_Nav_2_FD1,APIM_Request_Signals_1_FD1,APIM_Request_Signals_FD1,APIM_Send_Signals1_FD1,APIM_Send_Signals_2_FD1,ActiveFrontStrg_Stat2_FD1,ActiveFrontStrg_Stat_FD1,AllTerrainControlData_FD1,All_Terrain_Data_FD1,BCM_Lamp_Stat_FD1,BatteryCharge_Data2_FD1,Battery_Mgmt_24V_FD1,Battery_Mgmt_2_FD1,Battery_Mgmt_3_FD1,Battery_Mgmt_4_FD1,Battery_Traction_1_FD1,Battery_Traction_3_FD1,Battery_Traction_4_FD1,Battery_Traction_5_FD1,Battery_Traction_6_FD1,BodyInfo_3_FD1,Body_Info_10_FD1,Body_Info_4_FD1,Body_Info_6_FD1,Body_Info_8_FD1,Body_Info_9_FD1,Climate_Cntrl_Data_2_FD1,Climate_Control_Data_FD1,Cluster_Info1_FD1,Cluster_Info_3_FD1,Cluster_Lighting_Rq_FD1,Compressor_Req_FD1,CruiseCtrl_Strg_Data_FD1,DCACA_Data1_FD1,DCACA_Data2_FD1,DCACA_Data3_FD1,DifferentialCtrlData_1_FD1,Driver_Dr_Stat_FD1,Dsp_Request_Signals11_FD1,ElecHorizon_Data1_FD1,ElecHorizon_Data2_FD1,FourByFourSwitchData_FD1,Front_Distance_Req_FD1,GGCC_Config_Mgmt_ID_1_FD1,GWM_AutoSar_NetMgmt_FD1,GlobalClock_Data_FD1,Global_PATS_Cntrl_Info_FD1,IPC_Infotainment_FD1,IPC_Send_Signals_2_FD1,MHT_EV_Wakeup_FD1,Mc_Send_Signals_2_FD1,ParkAid_Aud_Warn_CmdM_FD1,Pass_Dr_Stat_FD1,Personality_APIM_Data_FD1,Personality_Data_FD1,Power_Liftgate_Stat_FD1,PreCond_Hev_Data1_FD1,PreCond_Hev_Data2_FD1,Suspension_Data_FD1,TesterPhysicalResGWM_FD1,TrailerAid_Data_FD1,TrailerAid_Stat1_FD1,TrailerAid_Stat2_FD1,TrailerBrakeInfo_FD1,TrailerInfo_2_FD1,TrailerInfo_FD1,VeyDynamics_Data_FD1
  wires:
  in_port/1 -> bus_selector/1  "Subsystem1"
  bus_selector/1 -> AC_Compressor_Data_FD1/1(in_port)  "<AC_Compressor_Data_FD1>"
  bus_selector/2 -> AC_Compressor_Req_FD1/1(in_port)  "<AC_Compressor_Req_FD1>"
  bus_selector/3 -> APIMGPS_Data_Nav_1_FD1/1(in_port)  "<APIMGPS_Data_Nav_1_FD1>"
  bus_selector/4 -> APIMGPS_Data_Nav_2_FD1/1(in_port)  "<APIMGPS_Data_Nav_2_FD1>"
  bus_selector/5 -> APIM_Request_Signals_1_FD1/1(in_port)  "<APIM_Request_Signals_1_FD1>"
  bus_selector/6 -> APIM_Request_Signals_FD1/1(in_port)  "<APIM_Request_Signals_FD1>"
  bus_selector/7 -> APIM_Send_Signals1_FD1/1(in_port)  "<APIM_Send_Signals1_FD1>"
  bus_selector/8 -> APIM_Send_Signals_2_FD1/1(in_port)  "<APIM_Send_Signals_2_FD1>"
  bus_selector/9 -> ActiveFrontStrg_Stat2_FD1/1(in_port)  "<ActiveFrontStrg_Stat2_FD1>"
  bus_selector/10 -> ActiveFrontStrg_Stat_FD1/1(in_port)  "<ActiveFrontStrg_Stat_FD1>"
  bus_selector/11 -> AllTerrainControlData_FD1/1(in_port)  "<AllTerrainControlData_FD1>"
  bus_selector/12 -> All_Terrain_Data_FD1/1(in_port)  "<All_Terrain_Data_FD1>"
  bus_selector/13 -> BCM_Lamp_Stat_FD1/1(in_port)  "<BCM_Lamp_Stat_FD1>"
  bus_selector/14 -> BatteryCharge_Data2_FD1/1(in_port)  "<BatteryCharge_Data2_FD1>"
  bus_selector/15 -> Battery_Mgmt_24V_FD1/1(in_port)  "<Battery_Mgmt_24V_FD1>"
  bus_selector/16 -> Battery_Mgmt_2_FD1/1(in_port)  "<Battery_Mgmt_2_FD1>"
  bus_selector/17 -> Battery_Mgmt_3_FD1/1(in_port)  "<Battery_Mgmt_3_FD1>"
  bus_selector/18 -> Battery_Mgmt_4_FD1/1(in_port)  "<Battery_Mgmt_4_FD1>"
  bus_selector/19 -> Battery_Traction_1_FD1/1(in_port)  "<Battery_Traction_1_FD1>"
  bus_selector/20 -> Battery_Traction_3_FD1/1(in_port)  "<Battery_Traction_3_FD1>"
  bus_selector/21 -> Battery_Traction_4_FD1/1(in_port)  "<Battery_Traction_4_FD1>"
  bus_selector/22 -> Battery_Traction_5_FD1/1(in_port)  "<Battery_Traction_5_FD1>"
  bus_selector/23 -> Battery_Traction_6_FD1/1(in_port)  "<Battery_Traction_6_FD1>"
  bus_selector/24 -> BodyInfo_3_FD1/1(in_port)  "<BodyInfo_3_FD1>"
  bus_selector/25 -> Body_Info_10_FD1/1(in_port)  "<Body_Info_10_FD1>"
  bus_selector/26 -> Body_Info_4_FD1/1(in_port)  "<Body_Info_4_FD1>"
  bus_selector/27 -> Body_Info_6_FD1/1(in_port)  "<Body_Info_6_FD1>"
  bus_selector/28 -> Body_Info_8_FD1/1(in_port)  "<Body_Info_8_FD1>"
  bus_selector/29 -> Body_Info_9_FD1/1(in_port)  "<Body_Info_9_FD1>"
  bus_selector/30 -> Climate_Cntrl_Data_2_FD1/1(in_port)  "<Climate_Cntrl_Data_2_FD1>"
  bus_selector/31 -> Climate_Control_Data_FD1/1(in_port)  "<Climate_Control_Data_FD1>"
  bus_selector/32 -> Cluster_Info1_FD1/1(in_port)  "<Cluster_Info1_FD1>"
  bus_selector/33 -> Cluster_Info_3_FD1/1(in_port)  "<Cluster_Info_3_FD1>"
  bus_selector/34 -> Cluster_Lighting_Rq_FD1/1(in_port)  "<Cluster_Lighting_Rq_FD1>"
  bus_selector/35 -> Compressor_Req_FD1/1(in_port)  "<Compressor_Req_FD1>"
  bus_selector/36 -> CruiseCtrl_Strg_Data_FD1/1(in_port)  "<CruiseCtrl_Strg_Data_FD1>"
  bus_selector/37 -> DCACA_Data1_FD1/1(in_port)  "<DCACA_Data1_FD1>"
  bus_selector/38 -> DCACA_Data2_FD1/1(in_port)  "<DCACA_Data2_FD1>"
  bus_selector/39 -> DCACA_Data3_FD1/1(in_port)  "<DCACA_Data3_FD1>"
  bus_selector/40 -> DifferentialCtrlData_1_FD1/1(in_port)  "<DifferentialCtrlData_1_FD1>"
  bus_selector/41 -> Driver_Dr_Stat_FD1/1(in_port)  "<Driver_Dr_Stat_FD1>"
  bus_selector/42 -> Dsp_Request_Signals11_FD1/1(in_port)  "<Dsp_Request_Signals11_FD1>"
  bus_selector/43 -> ElecHorizon_Data1_FD1/1(in_port)  "<ElecHorizon_Data1_FD1>"
  bus_selector/44 -> ElecHorizon_Data2_FD1/1(in_port)  "<ElecHorizon_Data2_FD1>"
  bus_selector/45 -> FourByFourSwitchData_FD1/1(in_port)  "<FourByFourSwitchData_FD1>"
  bus_selector/46 -> Front_Distance_Req_FD1/1(in_port)  "<Front_Distance_Req_FD1>"
  bus_selector/47 -> GGCC_Config_Mgmt_ID_1_FD1/1(in_port)  "<GGCC_Config_Mgmt_ID_1_FD1>"
  bus_selector/48 -> GWM_AutoSar_NetMgmt_FD1/1(in_port)  "<GWM_AutoSar_NetMgmt_FD1>"
  bus_selector/49 -> GlobalClock_Data_FD1/1(in_port)  "<GlobalClock_Data_FD1>"
  bus_selector/50 -> Global_PATS_Cntrl_Info_FD1/1(in_port)  "<Global_PATS_Cntrl_Info_FD1>"
  bus_selector/51 -> IPC_Infotainment_FD1/1(in_port)  "<IPC_Infotainment_FD1>"
  bus_selector/52 -> IPC_Send_Signals_2_FD1/1(in_port)  "<IPC_Send_Signals_2_FD1>"
  bus_selector/53 -> MHT_EV_Wakeup_FD1/1(in_port)  "<MHT_EV_Wakeup_FD1>"
  bus_selector/54 -> Mc_Send_Signals_2_FD1/1(in_port)  "<Mc_Send_Signals_2_FD1>"
  bus_selector/55 -> ParkAid_Aud_Warn_CmdM_FD1/1(in_port)  "<ParkAid_Aud_Warn_CmdM_FD1>"
  bus_selector/56 -> Pass_Dr_Stat_FD1/1(in_port)  "<Pass_Dr_Stat_FD1>"
  bus_selector/57 -> Personality_APIM_Data_FD1/1(in_port)  "<Personality_APIM_Data_FD1>"
  bus_selector/58 -> Personality_Data_FD1/1(in_port)  "<Personality_Data_FD1>"
  bus_selector/59 -> Power_Liftgate_Stat_FD1/1(in_port)  "<Power_Liftgate_Stat_FD1>"
  bus_selector/60 -> PreCond_Hev_Data1_FD1/1(in_port)  "<PreCond_Hev_Data1_FD1>"
  bus_selector/61 -> PreCond_Hev_Data2_FD1/1(in_port)  "<PreCond_Hev_Data2_FD1>"
  bus_selector/62 -> Suspension_Data_FD1/1(in_port)  "<Suspension_Data_FD1>"
  bus_selector/63 -> TesterPhysicalResGWM_FD1/1(in_port)  "<TesterPhysicalResGWM_FD1>"
  bus_selector/64 -> TrailerAid_Data_FD1/1(in_port)  "<TrailerAid_Data_FD1>"
  bus_selector/65 -> TrailerAid_Stat1_FD1/1(in_port)  "<TrailerAid_Stat1_FD1>"
  bus_selector/66 -> TrailerAid_Stat2_FD1/1(in_port)  "<TrailerAid_Stat2_FD1>"
  bus_selector/67 -> TrailerBrakeInfo_FD1/1(in_port)  "<TrailerBrakeInfo_FD1>"
  bus_selector/68 -> TrailerInfo_2_FD1/1(in_port)  "<TrailerInfo_2_FD1>"
  bus_selector/69 -> TrailerInfo_FD1/1(in_port)  "<TrailerInfo_FD1>"
  bus_selector/70 -> VeyDynamics_Data_FD1/1(in_port)  "<VeyDynamics_Data_FD1>"

== system P702_NI_SoftECU/Output/Subsystem1/CAN_Signal/GWM/RCM ==
  in_port : Inport
  RCMSerialNumber_FD1_454 : Subsystem
  RCMStatusMessage2_FD1_4C : Subsystem
  bus_selector : BusSelector  OutputSignals=RCMStatusMessage2_FD1_4C,RCMSerialNumber_FD1_454
  wires:
  in_port/1 -> bus_selector/1  "Subsystem1"
  bus_selector/1 -> RCMStatusMessage2_FD1_4C/1(in_port)  "<RCMStatusMessage2_FD1_4C>"
  bus_selector/2 -> RCMSerialNumber_FD1_454/1(in_port)  "<RCMSerialNumber_FD1_454>"

== system P702_NI_SoftECU/Output/Subsystem1/CAN_Signal/GWM/SCCM ==
  in_port : Inport
  Steering_Data_FD1_83 : Subsystem
  Steering_Wheel_Data2_FD1_81 : Subsystem
  bus_selector : BusSelector  OutputSignals=Steering_Data_FD1_83,Steering_Wheel_Data2_FD1_81
  wires:
  in_port/1 -> bus_selector/1  "Subsystem1"
  bus_selector/1 -> Steering_Data_FD1_83/1(in_port)  "<Steering_Data_FD1_83>"
  bus_selector/2 -> Steering_Wheel_Data2_FD1_81/1(in_port)  "<Steering_Wheel_Data2_FD1_81>"

== system P702_NI_SoftECU/Output/Subsystem1/CAN_Signal/GWM/Tester//AutoSar ==
  in_port : Inport
  GWM_AutoSar_NetMgmt_FD1 : Subsystem
  TesterPhysicalResGWM_FD1 : Subsystem
  bus_selector : BusSelector  OutputSignals=GWM_AutoSar_NetMgmt_FD1,TesterPhysicalResGWM_FD1
  wires:
  in_port/1 -> bus_selector/1  "Subsystem1"
  bus_selector/1 -> GWM_AutoSar_NetMgmt_FD1/1(in_port)  "<GWM_AutoSar_NetMgmt_FD1>"
  bus_selector/2 -> TesterPhysicalResGWM_FD1/1(in_port)  "<TesterPhysicalResGWM_FD1>"

== system P702_NI_SoftECU/Output/Subsystem1/CAN_Signal/PSCM/EPAS_INFO_0x82 ==
  in_port : Inport
  DrvSteActv_B_Stat : Terminator
  DrvSte_Tq_Actl : Terminator
  EPAS_Failure : Terminator
  SAPPAngleControlStat{1..6} (6 alike) : Terminator
  SteMdule_D_Stat : Terminator
  SteMdule_I_Est : Terminator
  SteMdule_U_Meas : Terminator
  SteeringColumnTorque : Terminator
  TrlrHitchLamp_D_Rqst : Terminator
  VehVTrlrAid_B_Rq : Terminator
  Veh_V_RqMxTrlrAid : Terminator
  bus_selector : BusSelector  OutputSignals=SteeringColumnTorque,SAPPAngleControlStat6,SAPPAngleControlStat5,SAPPAngleControlStat4,SAPPAngleControlStat3,SAPPAngleControlStat2,DrvSteActv_B_Stat,EPAS_Failure,SAPPAngleControlStat1,SteMdule_I_Est,VehVTrlrAid_B_Rq,TrlrHitchLamp_D_Rqst,SteMdule_U_Meas,DrvSte_Tq_Actl,SteMdule_D_Stat,Veh_V_RqMxTrlrAid
  wires:
  in_port/1 -> bus_selector/1  "Subsystem1"
  bus_selector/1 -> SteeringColumnTorque/1  "<SteeringColumnTorque>"
  bus_selector/2 -> SAPPAngleControlStat6/1  "<SAPPAngleControlStat6>"
  bus_selector/3 -> SAPPAngleControlStat5/1  "<SAPPAngleControlStat5>"
  bus_selector/4 -> SAPPAngleControlStat4/1  "<SAPPAngleControlStat4>"
  bus_selector/5 -> SAPPAngleControlStat3/1  "<SAPPAngleControlStat3>"
  bus_selector/6 -> SAPPAngleControlStat2/1  "<SAPPAngleControlStat2>"
  bus_selector/7 -> DrvSteActv_B_Stat/1  "<DrvSteActv_B_Stat>"
  bus_selector/8 -> EPAS_Failure/1  "<EPAS_Failure>"
  bus_selector/9 -> SAPPAngleControlStat1/1  "<SAPPAngleControlStat1>"
  bus_selector/10 -> SteMdule_I_Est/1  "<SteMdule_I_Est>"
  bus_selector/11 -> VehVTrlrAid_B_Rq/1  "<VehVTrlrAid_B_Rq>"
  bus_selector/12 -> TrlrHitchLamp_D_Rqst/1  "<TrlrHitchLamp_D_Rqst>"
  bus_selector/13 -> SteMdule_U_Meas/1  "<SteMdule_U_Meas>"
  bus_selector/14 -> DrvSte_Tq_Actl/1  "<DrvSte_Tq_Actl>"
  bus_selector/15 -> SteMdule_D_Stat/1  "<SteMdule_D_Stat>"
  bus_selector/16 -> Veh_V_RqMxTrlrAid/1  "<Veh_V_RqMxTrlrAid>"

== system P702_NI_SoftECU/Output/Subsystem1/CAN_Signal/PSCM/Lane_Assist_Data3_FD1_0x3CC ==
  in_port : Inport
  LaActAvail_D_Actl : Terminator
  LaActDeny_B_Actl : Terminator
  LaHandsOff_B_Actl : Terminator
  LsmcBrkDecelEnbl_D_Rq : Terminator
  LsmcBrk_Tq_Rq : Terminator
  TjaHandsOnCnfdnc_B_Est : Terminator
  TrlrAn_An_TrgtCalc : Terminator
  bus_selector : BusSelector  OutputSignals=LaHandsOff_B_Actl,LaActDeny_B_Actl,LaActAvail_D_Actl,TjaHandsOnCnfdnc_B_Est,LsmcBrkDecelEnbl_D_Rq,LsmcBrk_Tq_Rq,TrlrAn_An_TrgtCalc
  wires:
  in_port/1 -> bus_selector/1  "Subsystem1"
  bus_selector/1 -> LaHandsOff_B_Actl/1  "<LaHandsOff_B_Actl>"
  bus_selector/2 -> LaActDeny_B_Actl/1  "<LaActDeny_B_Actl>"
  bus_selector/3 -> LaActAvail_D_Actl/1  "<LaActAvail_D_Actl>"
  bus_selector/4 -> TjaHandsOnCnfdnc_B_Est/1  "<TjaHandsOnCnfdnc_B_Est>"
  bus_selector/5 -> LsmcBrkDecelEnbl_D_Rq/1  "<LsmcBrkDecelEnbl_D_Rq>"
  bus_selector/6 -> LsmcBrk_Tq_Rq/1  "<LsmcBrk_Tq_Rq>"
  bus_selector/7 -> TrlrAn_An_TrgtCalc/1  "<TrlrAn_An_TrgtCalc>"

== system P702_NI_SoftECU/Output/Subsystem1/CAN_Signal/PSCM/PSCM_AutoSar_NetwrkMgmt_0x5B5 ==
  in_port : Inport
  PSCM_AutoSarNMControl : Terminator
  PSCM_AutoSarNMNodeId : Terminator
  PSCM_AutoSarNMReserved{1..4} (4 alike) : Terminator
  PSCM_GWNMProxy : Terminator
  PSCM_GWOnBoardTester : Terminator
  bus_selector : BusSelector  OutputSignals=PSCM_AutoSarNMNodeId,PSCM_AutoSarNMControl,PSCM_AutoSarNMReserved1,PSCM_AutoSarNMReserved2,PSCM_GWOnBoardTester,PSCM_GWNMProxy,PSCM_AutoSarNMReserved3,PSCM_AutoSarNMReserved4
  wires:
  in_port/1 -> bus_selector/1  "Subsystem1"
  bus_selector/1 -> PSCM_AutoSarNMNodeId/1  "<PSCM_AutoSarNMNodeId>"
  bus_selector/2 -> PSCM_AutoSarNMControl/1  "<PSCM_AutoSarNMControl>"
  bus_selector/3 -> PSCM_AutoSarNMReserved1/1  "<PSCM_AutoSarNMReserved1>"
  bus_selector/4 -> PSCM_AutoSarNMReserved2/1  "<PSCM_AutoSarNMReserved2>"
  bus_selector/5 -> PSCM_GWOnBoardTester/1  "<PSCM_GWOnBoardTester>"
  bus_selector/6 -> PSCM_GWNMProxy/1  "<PSCM_GWNMProxy>"
  bus_selector/7 -> PSCM_AutoSarNMReserved3/1  "<PSCM_AutoSarNMReserved3>"
  bus_selector/8 -> PSCM_AutoSarNMReserved4/1  "<PSCM_AutoSarNMReserved4>"

== system P702_NI_SoftECU/Output/Subsystem1/CAN_Signal/PSCM/SteeringPinion_Data_0x7E ==
  in_port : Inport
  StePinAn_No_Cnt : Terminator
  StePinAn_No_Cs : Terminator
  StePinCompAnEst_D_Qf : Terminator
  StePinComp_An_Est : Terminator
  StePinRelInit_An_Sns : Terminator
  StePw_B_Rq : Terminator
  bus_selector : BusSelector  OutputSignals=StePinRelInit_An_Sns,StePw_B_Rq,StePinComp_An_Est,StePinAn_No_Cs,StePinAn_No_Cnt,StePinCompAnEst_D_Qf
  wires:
  in_port/1 -> bus_selector/1  "Subsystem1"
  bus_selector/1 -> StePinRelInit_An_Sns/1  "<StePinRelInit_An_Sns>"
  bus_selector/2 -> StePw_B_Rq/1  "<StePw_B_Rq>"
  bus_selector/3 -> StePinComp_An_Est/1  "<StePinComp_An_Est>"
  bus_selector/4 -> StePinAn_No_Cs/1  "<StePinAn_No_Cs>"
  bus_selector/5 -> StePinAn_No_Cnt/1  "<StePinAn_No_Cnt>"
  bus_selector/6 -> StePinCompAnEst_D_Qf/1  "<StePinCompAnEst_D_Qf>"

== system P702_NI_SoftECU/Output/Subsystem1/CAN_Signal/PSCM/TesterPhysicalResPSCM_0x738 ==
  in_port : Inport
  TesterPhysicalResPSCM : Terminator
  bus_selector : BusSelector  OutputSignals=TesterPhysicalResPSCM
  wires:
  in_port/1 -> bus_selector/1  "Subsystem1"
  bus_selector/1 -> TesterPhysicalResPSCM/1  "<TesterPhysicalResPSCM>"

== system P702_NI_SoftECU/Output/Subsystem1/CAN_Signal/PSCM/TrailerAid_Data2_0x417 ==
  in_port : Inport
  EsaOn_B_Stat : Terminator
  HitchToTrlrAxle_L_Calc : Terminator
  LatCtlLim_D_Stat : Terminator
  LatCtlSte_D_Stat : Terminator
  SelDrvMdeSte_D_Stat : Terminator
  TrlrAidEnbl_D2_Stat : Terminator
  TrlrAidMsgTxt_D2_Rq : Terminator
  TrlrAidSetup_D2_Stat : Terminator
  TrlrAidTrgtId_No_Rq : Terminator
  TrlrAidTrlrId_No_Rq : Terminator
  TrlrAnOffst_An2_Calc : Terminator
  TrlrAn_An_MxCalc : Terminator
  TrlrAn_An_WarnCalc : Terminator
  bus_selector : BusSelector  OutputSignals=HitchToTrlrAxle_L_Calc,TrlrAidMsgTxt_D2_Rq,EsaOn_B_Stat,LatCtlLim_D_Stat,LatCtlSte_D_Stat,SelDrvMdeSte_D_Stat,TrlrAidEnbl_D2_Stat,TrlrAn_An_WarnCalc,TrlrAnOffst_An2_Calc,TrlrAidSetup_D2_Stat,TrlrAidTrgtId_No_Rq,TrlrAn_An_MxCalc,TrlrAidTrlrId_No_Rq
  wires:
  in_port/1 -> bus_selector/1  "Subsystem1"
  bus_selector/1 -> HitchToTrlrAxle_L_Calc/1  "<HitchToTrlrAxle_L_Calc>"
  bus_selector/2 -> TrlrAidMsgTxt_D2_Rq/1  "<TrlrAidMsgTxt_D2_Rq>"
  bus_selector/3 -> EsaOn_B_Stat/1  "<EsaOn_B_Stat>"
  bus_selector/4 -> LatCtlLim_D_Stat/1  "<LatCtlLim_D_Stat>"
  bus_selector/5 -> LatCtlSte_D_Stat/1  "<LatCtlSte_D_Stat>"
  bus_selector/6 -> SelDrvMdeSte_D_Stat/1  "<SelDrvMdeSte_D_Stat>"
  bus_selector/7 -> TrlrAidEnbl_D2_Stat/1  "<TrlrAidEnbl_D2_Stat>"
  bus_selector/8 -> TrlrAn_An_WarnCalc/1  "<TrlrAn_An_WarnCalc>"
  bus_selector/9 -> TrlrAnOffst_An2_Calc/1  "<TrlrAnOffst_An2_Calc>"
  bus_selector/10 -> TrlrAidSetup_D2_Stat/1  "<TrlrAidSetup_D2_Stat>"
  bus_selector/11 -> TrlrAidTrgtId_No_Rq/1  "<TrlrAidTrgtId_No_Rq>"
  bus_selector/12 -> TrlrAn_An_MxCalc/1  "<TrlrAn_An_MxCalc>"
  bus_selector/13 -> TrlrAidTrlrId_No_Rq/1  "<TrlrAidTrlrId_No_Rq>"

== system P702_NI_SoftECU/Output/Subsystem1/CAN_Signal/RealPCM/EngBrakeData ==
  in_port : Inport
  CcStat_D_Actl : Terminator
  bus_selector : BusSelector  OutputSignals=CcStat_D_Actl
  wires:
  in_port/1 -> bus_selector/1  "Subsystem1"
  bus_selector/1 -> CcStat_D_Actl/1  "<CcStat_D_Actl>"

== system P702_NI_SoftECU/Output/Subsystem1/CAN_Signal/RealPCM/EngVehicleSpThrottle2 ==
  in_port : Inport
  Veh_V_ActlEng : Terminator
  bus_selector : BusSelector  OutputSignals=Veh_V_ActlEng
  wires:
  in_port/1 -> bus_selector/1  "Subsystem1"
  bus_selector/1 -> Veh_V_ActlEng/1  "<Veh_V_ActlEng>"

== system P702_NI_SoftECU/Output/Subsystem1/CAN_Signal/RealPCM/user_channel ==
  in_port : Inport
  Desired_Speed : Terminator
  PCM_status_user_input : Terminator
  bus_selector : BusSelector  OutputSignals=PCM_status_user_input,Desired_Speed
  wires:
  in_port/1 -> bus_selector/1  "Subsystem1"
  bus_selector/1 -> PCM_status_user_input/1  "<PCM_status_user_input>"
  bus_selector/2 -> Desired_Speed/1  "<Desired_Speed>"

== system P702_NI_SoftECU/Output/Subsystem1/To_NI_HIL/DSMC/DrvStatMonData ==
  in_port : Inport
  DrvEngLvlConfid_D_Stat : Terminator
  DrvEngageLevel_No_Cnt : Terminator
  DrvEngageLevel_No_Cs : Terminator
  bus_selector : BusSelector  OutputSignals=DrvEngLvlConfid_D_Stat,DrvEngageLevel_No_Cs,DrvEngageLevel_No_Cnt
  wires:
  in_port/1 -> bus_selector/1  "Subsystem1"
  bus_selector/1 -> DrvEngLvlConfid_D_Stat/1  "<DrvEngLvlConfid_D_Stat>"
  bus_selector/2 -> DrvEngageLevel_No_Cs/1  "<DrvEngageLevel_No_Cs>"
  bus_selector/3 -> DrvEngageLevel_No_Cnt/1  "<DrvEngageLevel_No_Cnt>"

== system P702_NI_SoftECU/Output/Subsystem1/To_NI_HIL/SRR_L/FL_SOD ==
  in_port : Inport
  SRR_FL_001 : Subsystem
  SRR_FL_002 : Subsystem
  SRR_FL_003 : Subsystem
  bus_selector : BusSelector  OutputSignals=SRR_FL_001,SRR_FL_002,SRR_FL_003
  wires:
  in_port/1 -> bus_selector/1  "Subsystem1"
  bus_selector/1 -> SRR_FL_001/1(in_port)  "<SRR_FL_001>"
  bus_selector/2 -> SRR_FL_002/1(in_port)  "<SRR_FL_002>"
  bus_selector/3 -> SRR_FL_003/1(in_port)  "<SRR_FL_003>"

== system P702_NI_SoftECU/Output/Subsystem1/To_NI_HIL/SRR_L/RL_SOD ==
  in_port : Inport
  SRR_RL_001 : Subsystem
  SRR_RL_002 : Subsystem
  SRR_RL_003 : Subsystem
  bus_selector : BusSelector  OutputSignals=SRR_RL_001,SRR_RL_002,SRR_RL_003
  wires:
  in_port/1 -> bus_selector/1  "Subsystem1"
  bus_selector/1 -> SRR_RL_001/1(in_port)  "<SRR_RL_001>"
  bus_selector/2 -> SRR_RL_002/1(in_port)  "<SRR_RL_002>"
  bus_selector/3 -> SRR_RL_003/1(in_port)  "<SRR_RL_003>"

== system P702_NI_SoftECU/Output/Subsystem1/To_NI_HIL/SRR_R/FR_SOD ==
  in_port : Inport
  SRR_FR_001 : Subsystem
  SRR_FR_002 : Subsystem
  SRR_FR_003 : Subsystem
  bus_selector : BusSelector  OutputSignals=SRR_FR_001,SRR_FR_002,SRR_FR_003
  wires:
  in_port/1 -> bus_selector/1  "Subsystem1"
  bus_selector/1 -> SRR_FR_001/1(in_port)  "<SRR_FR_001>"
  bus_selector/2 -> SRR_FR_002/1(in_port)  "<SRR_FR_002>"
  bus_selector/3 -> SRR_FR_003/1(in_port)  "<SRR_FR_003>"

== system P702_NI_SoftECU/Output/Subsystem1/To_NI_HIL/SRR_R/RR_SOD ==
  in_port : Inport
  SRR_RR_001 : Subsystem
  SRR_RR_002 : Subsystem
  SRR_RR_003 : Subsystem
  bus_selector : BusSelector  OutputSignals=SRR_RR_001,SRR_RR_002,SRR_RR_003
  wires:
  in_port/1 -> bus_selector/1  "Subsystem1"
  bus_selector/1 -> SRR_RR_001/1(in_port)  "<SRR_RR_001>"
  bus_selector/2 -> SRR_RR_002/1(in_port)  "<SRR_RR_002>"
  bus_selector/3 -> SRR_RR_003/1(in_port)  "<SRR_RR_003>"
